simulink model "g_s_cl_old"  (Simulink 5.0)
settings: Solver=ode45  StartTime=0.0  StopTime=10.0  RelTol=1e-3
values from neighbouring files (symbols this model uses):
  D1 = D    [tfvar.m]
undefined symbols (not defined in the file or in its folder): D2, den, N1, N2, N_var, num, R, S, st, T, tau, Ts
settings Model: Creator=kannan  LastModifiedBy=kannan  ExtModeAutoUpdateStatusClock=off

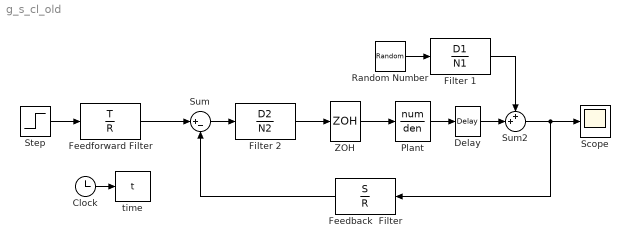
== system g_s_cl_old ==
  " Filter 2" : DiscreteFilter  Numerator=D2  Denominator=N2  SampleTime=Ts
  Clock : Clock
      settings: Decimation=10
  Delay : TransportDelay  DelayTime=tau
  Feedback  Filter : DiscreteFilter  Orientation=left  Numerator=S  Denominator=R  SampleTime=Ts
  Feedforward Filter : DiscreteFilter  Numerator=T  Denominator=R  SampleTime=Ts
  Filter 1 : DiscreteFilter  Numerator=D1  Denominator=N1  SampleTime=Ts
  Plant : TransferFcn  Numerator=num  Denominator=den
  Random Number : RandomNumber  Variance=N_var  SampleTime=Ts
  Scope : Scope
      settings: YMin=-6e+164  YMax=1.02293e+149
  Step : Step  Time=0  After=st  SampleTime=Ts
  Sum : Sum  Inputs=|+-  SaturateOnIntegerOverflow=on
  Sum2 : Sum  Inputs=++|  SaturateOnIntegerOverflow=on
  ZOH : ZeroOrderHold  SampleTime=Ts
  time : ToWorkspace  VariableName=t  SampleTime=Ts  SaveFormat=Array
  wires:
  Step/1 -> Feedforward Filter/1
  Feedforward Filter/1 -> Sum/1
  Feedback  Filter/1 -> Sum/2
  Clock/1 -> time/1
  Filter 1/1 -> Sum2/1
  Random Number/1 -> Filter 1/1
  Sum2/1 -> Scope/1, Feedback  Filter/1
  Sum/1 -> " Filter 2"/1
  Plant/1 -> Delay/1
  " Filter 2"/1 -> ZOH/1
  ZOH/1 -> Plant/1
  Delay/1 -> Sum2/2
